simulink model "drone_stud2018"  (R2024b)
settings: Solver=FixedStepAuto  StartTime=0.0  StopTime=100  FixedStep=0.001  RelTol=1e-3
values from neighbouring files (symbols this model uses):
  K = place(A, B, p)    [drone_param_stud.m]
  Ki = [0   0  Kiz ... (first row only)    [drone_param_stud.m]
settings Model: Creator=zigg  LastModifiedBy=acldpr
settings SolverCC: AlgebraicLoopSolver=TrustRegion
settings DataIOCC: ReturnWorkspaceOutputs=off
settings DebuggingCC: UnconnectedInputMsg=warning  UnconnectedOutputMsg=warning  UnconnectedLineMsg=warning  ArithmeticOperatorsInVariantConditions=warning
settings ModelReferenceCC: EnableRefExpFcnMdlSchedulingChecks=on
settings SFSimCC: SimUseLocalCustomCode=off  CustomCodeUndefinedFunction=UseInterfaceOnly
settings RTWCC: RTWUseLocalCustomCode=off  GPUComputeCapability=3.5
settings CodeAppCC: StateflowObjectComments=on

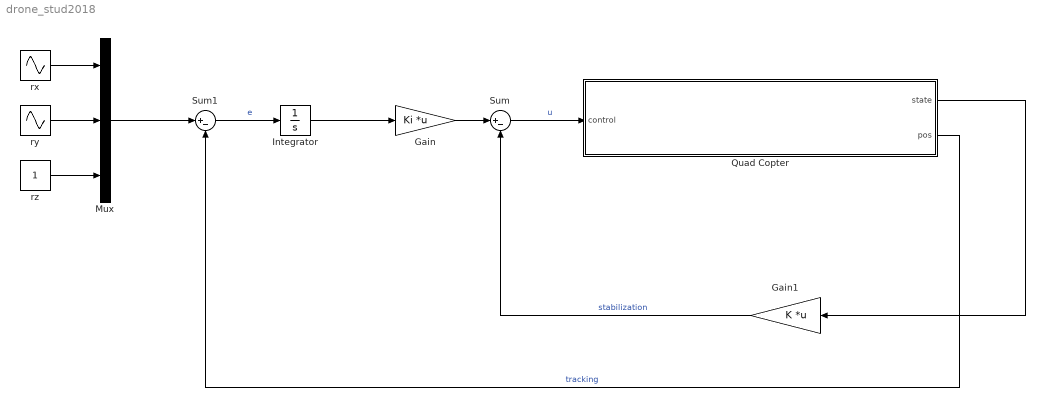
== system drone_stud2018 ==
  Gain : Gain  Gain=Ki  Multiplication=Matrix(K*u)
  Gain1 : Gain  Gain=K  Multiplication=Matrix(K*u)
  Integrator : Integrator
  Mux : Mux  Inputs=3
  Quad Copter : Subsystem
  Sum : Sum  Inputs=|+-
  Sum1 : Sum  Inputs=|+-
  rx : Sin  SampleTime=0
  ry : Sin  Phase=pi/2  SampleTime=0
  rz : Constant
  wires:
  Sum/1 -> Quad Copter/1(control)  "u"
  Gain/1 -> Sum/1
  Sum1/1 -> Integrator/1  "e"
  Integrator/1 -> Gain/1
  Gain1/1 -> Sum/2  "stabilization"
  Quad Copter/2(pos) -> Sum1/2  "tracking"
  Quad Copter/1(state) -> Gain1/1
  Mux/1 -> Sum1/1
  ry/1 -> Mux/2
  rx/1 -> Mux/1
  rz/1 -> Mux/3

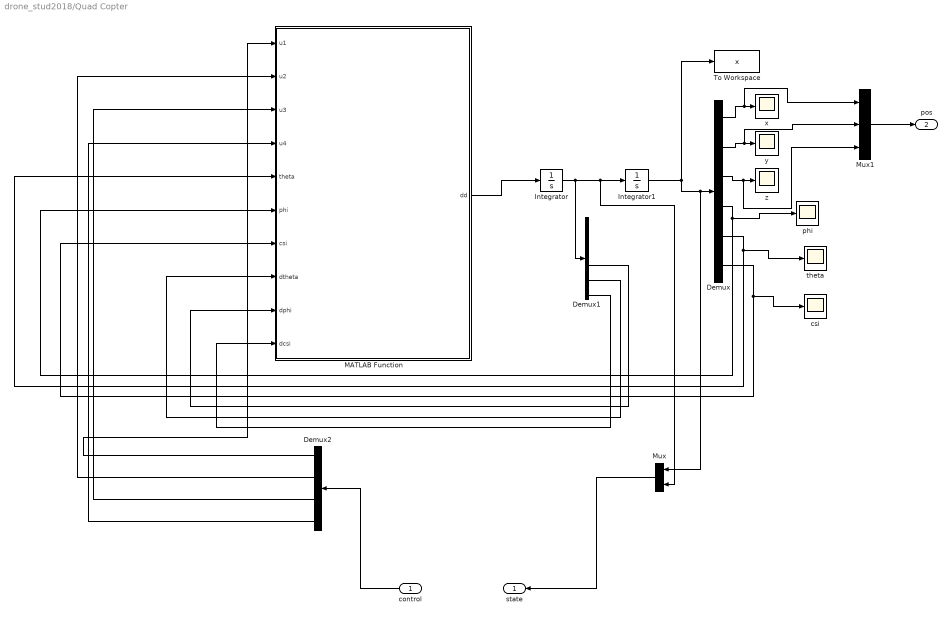
== system drone_stud2018/Quad Copter ==
  control : Inport  PortDimensions=4
  Demux : Demux  Outputs=6
  Demux1 : Demux  Outputs=6
  Demux2 : Demux
  Integrator : Integrator
  Integrator1 : Integrator  InitialCondition=[0.1 0.2 0.3 0 0 0.1]
  MATLAB Function : MATLAB Function  TreatAsAtomicUnit=on
  Mux : Mux  Inputs=2
      settings: DisplayOption=signals
  Mux1 : Mux  Inputs=3
  To Workspace : ToWorkspace  VariableName=x  SampleTime=-1
  csi : Scope
  phi : Scope
  theta : Scope
  x : Scope
  y : Scope
  z : Scope
  state : Outport
  pos : Outport  Port=2
  wires:
  Integrator/1 -> Demux1/1, Mux/2, Integrator1/1
  MATLAB Function/1(dd) -> Integrator/1
  Integrator1/1 -> Mux/1, Demux/1, To Workspace/1
  Demux/1 -> Mux1/1, x/1
  Demux/2 -> Mux1/2, y/1
  Demux/3 -> Mux1/3, z/1
  Demux/4 -> phi/1, MATLAB Function/6(phi)
  Demux/5 -> theta/1, MATLAB Function/5(theta)
  Demux/6 -> csi/1, MATLAB Function/7(csi)
  Demux1/4 -> MATLAB Function/9(dphi)
  Demux1/5 -> MATLAB Function/8(dtheta)
  Demux1/6 -> MATLAB Function/10(dcsi)
  Mux/1 -> state/1
  Demux2/1 -> MATLAB Function/1(u1)
  Demux2/2 -> MATLAB Function/2(u2)
  Demux2/3 -> MATLAB Function/3(u3)
  Demux2/4 -> MATLAB Function/4(u4)
  control/1 -> Demux2/1
  Mux1/1 -> pos/1

== matlab function drone_stud2018/Quad Copter/MATLAB Function ==
  data: u1 input; u2 input; u3 input; u4 input; dd output; theta input; phi input; csi input; dtheta input; dphi input; dcsi input
function dd = fcn( u1,u2,u3,u4, theta, phi, csi, dtheta, dphi, dcsi)

m=0.4;
Ix=0.002;
Iy=0.0016;
Iz=0.0035;
b=192.32*10^(-7);
d=1*10^(-7);
l=0.1778;
g=9.8;
c=1.9712;

J=[Ix 0 -Ix*sin(theta);
     0  Iy*(cos(phi))^2+Iz*(sin(phi))^2     (Iy-Iz)*cos(phi)*sin(phi)*cos(theta);
     -Ix*sin(theta)  (Iy-Iz)*cos(phi)*sin(phi)*cos(theta)   Ix*(sin(theta))^2+Iy*(sin(phi))^2*(cos(theta))^2+Iz*(cos(phi))^2*(cos(theta))^2];
 
 c11=0;
 c12=(Iy-Iz)*(dtheta*cos(phi)*sin(phi)+dphi*(sin(phi))^2*cos(theta))+(Iz-Iy)*dcsi*(cos(phi))^2*cos(theta)-Ix*dcsi*cos(theta);
 c13=(Iz-Iy)*dcsi*(cos(theta))^2*sin(phi)*cos(phi);
 c21=(Iz-Iy)*(dtheta*sin(phi)*cos(phi)+dphi*(sin(phi))^2*cos(theta))+(Iy-Iz)*dcsi*(cos(phi))^2*cos(theta)+Ix*dcsi*cos(theta);
 c22=(Iz-Iy)*dphi*cos(phi)*sin(phi);
 c23=-Ix*dcsi*sin(theta)*cos(theta)+Iy*dcsi*(sin(phi))^2*sin(theta)*cos(theta)+Iz*dcsi*(cos(phi))^2*sin(theta)*cos(theta);
 c31=(Iy-Iz)*dcsi*(cos(theta))^2*sin(phi)*cos(phi)-Ix*dtheta*cos(theta);
 c32=(Iz-Iy)*(dtheta*cos(phi)*sin(phi)*sin(theta)+dphi*(sin(phi))^2*cos(theta))+(Iy-Iz)*dphi*(cos(phi))^2*cos(theta)+Ix*dcsi*sin(theta)*cos(theta)-Iy*dcsi*(sin(phi))^2*sin(theta)*cos(theta)-Iz*dcsi*(cos(phi))^2*sin(theta)*cos(theta);
 c33=(Iy-Iz)*dphi*(cos(theta))^2*sin(phi)*cos(phi)-Iy*dtheta*(sin(phi))^2*sin(theta)*cos(theta)-Iz*dtheta*(cos(phi))^2*sin(theta)*cos(theta)+Ix*dtheta*sin(theta)*cos(theta);
 
 C=[c11 c12 c13;c21 c22 c23; c31 c32 c33];
 
 Jinv=inv(J);
 
 Utheta=u3;
 Uphi=u2; 
 Ucsi=u4;
 Ucoll=u1+m*g;
 
 %Ucoll=m*g+delta_Ucoll;
 
 %F1=b*c^2*u1^2;F2=b*c^2*u2^2;F3=b*c^2*u3^2;F4=b*c^2*u4^2;
 %tau1=d*c^2*u1^2;tau2=d*c^2*u2^2;tau3=d*c^2*u3^2;tau4=d*c^2*u4^2;
 
 %Ucol=F1+F2+F3+F4;
 %Uphi=l*(F1-F3);
 %Utheta=l*(-F4+F2);
 %Ucsi=tau1+tau3-tau2-tau4;
 
 ddx=(cos(phi)*sin(theta)*cos(csi)+sin(phi)*sin(csi))*Ucoll/m;
 ddy=(cos(phi)*sin(theta)*sin(csi)-sin(phi)*cos(csi))*Ucoll/m;
 ddz=-g+cos(phi)*cos(theta)*Ucoll/m;
 ddangle=Jinv*([Uphi;Utheta;Ucsi]-C*[dphi;dtheta;dcsi]);
 ddphi=ddangle(1);
 ddtheta=ddangle(2);
 ddcsi=ddangle(3);
  
 dd=[ddx;ddy;ddz;ddphi;ddtheta;ddcsi];
